simulink model "DogGait_Sine"  (R2022b)
settings: Solver=FixedStepAuto  StartTime=0.0  StopTime=inf  RelTol=1e-3
undefined symbols (not defined in the file): C, D, f
libraries: vexv5lib x24, vexcommonlib x16, Vex_V5_Simulink_Expansion x8
settings Model: Creator=Serious Chimp  LastModifiedBy=Serious Chimp
settings DataIOCC: SaveFormat=StructureWithTime  InspectSignalLogs=on
settings OptimizationCC: EnhancedBackFolding=on  PassReuseOutputArgsAs=Individual arguments  ZeroExternalMemoryAtStartup=off  ZeroInternalMemoryAtStartup=off  MaxStackSize=64  OptimizeBlockOrder=speed  DifferentSizesBufferReuse=on  OptimizationCustomize=off  EfficientTunableParamExpr=on
settings DebuggingCC: ParameterTunabilityLossMsg=error
settings HardwareCC: ProdBitPerPointer=32  ProdBitPerSizeT=32  ProdBitPerPtrDiffT=32  ProdLargestAtomicInteger=Long  ProdLargestAtomicFloat=Double  ProdWordSize=32  ProdHWDeviceType=ARM Compatible->ARM Cortex  UseEmbeddedCoderFeatures=off
settings SFSimCC: MATLABDynamicMemAlloc=off
settings RTWCC: Description=Embedded Coder  SystemTargetFile=ert.tlc  HardwareBoard=VEX V5 Robot Brain  TLCOptions="-aInlineSetEventsForThisBaseRateFcn=TLC_FALSE -aSuppressMultiTaskScheduler=TLC_FALSE  -aRateBasedStepFcn=0"  TemplateMakefile=ert_default_tmf  Toolchain=GNU Tools for ARM Embedded Processors
settings CodeAppCC: ForceParamTrailComments=on  IgnoreCustomStorageClasses=off  OperatorAnnotations=on  SimulinkDataObjDesc=on  SFDataObjDesc=on  InsertBlockDesc=on
settings ERTTargetCC: SupportNonInlinedSFcns=on  ExtModeTransport=3  ExtModeStaticAlloc=on  ExtModeStaticAllocSize=2048  ExtModeMexFile=ext_xcp  ExtModeIntrfLevel=Level2 - Open

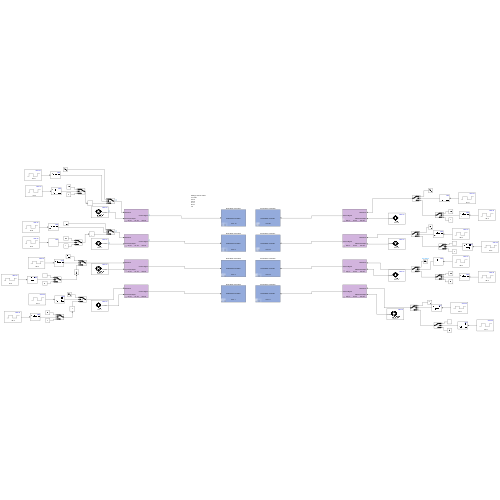
[thumbnail: Simulink's stored preview of the top-level diagram]
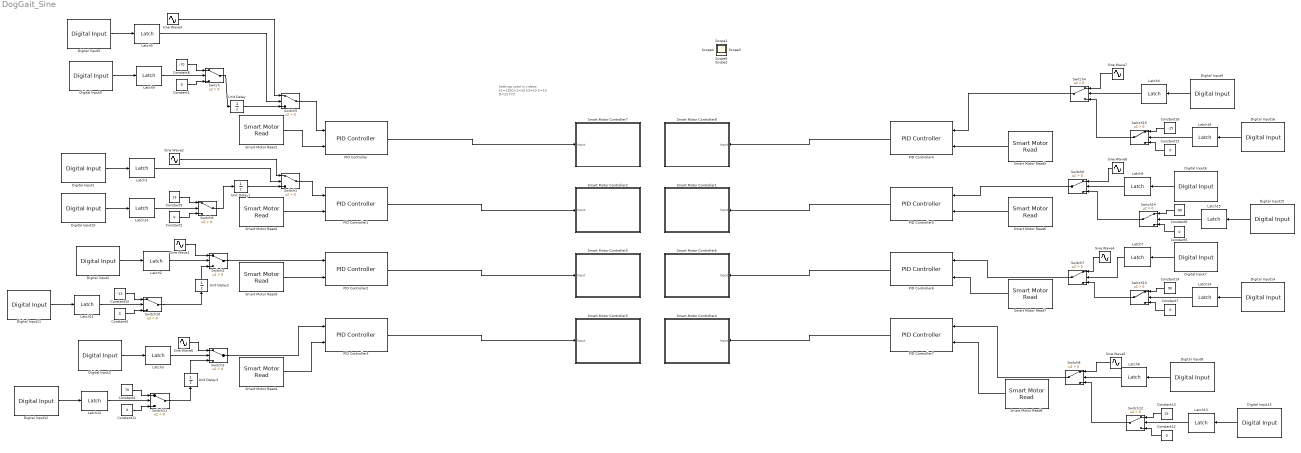
== system DogGait_Sine ==
  note: Settings used in videos:
      | k1=1200
      | k2=10
      | k3=10
      | C=15
      | D=23
      | f=5
  Constant{1..3,5,7,11..12,15} (8 alike) : Constant  Value=0
  Constant10 : Constant  Value=-13
  Constant13 : Constant  Value=15
  Constant14 : Constant  Value=90
  Constant16 : Constant  Value=-15
  Constant4 : Constant  Value=70
  Constant6 : Constant  Value=-90
  Constant8 : Constant  Value=-70
  Constant9 : Constant  Value=13
  Digital Input{1..8} (8 alike) : vexv5lib/Sensors/Digital Input  smartPort3wire=None  port=H  SampleTime=0.2
  Digital Input{9..16} (8 alike) : vexv5lib/Sensors/Digital Input  smartPort3wire=None  port=A  SampleTime=0.2
  Latch{1..16} (16 alike) : vexcommonlib/Latch  output0=off  BlockPlatform=vexv5
      settings: LibrarySourceBlock=vexv5lib/Utilities/Latch
  PID Controller : Vex_V5_Simulink_Expansion/Core Blocks/PID Controller  KP=k1  KI=k3  KD=k2  LimitOutput=off  limitHigh=10  limitLow=10  AntiWindupMode=none  kb=0
      settings: SourceProductName=Vex V5 Simulink Expansion
  PID Controller{1..7} (7 alike) : Vex_V5_Simulink_Expansion/Core Blocks/PID Controller  KP=k1  KI=k3  KD=k2  LimitOutput=off  limitHigh=0  limitLow=0  AntiWindupMode=none  kb=0
      settings: SourceProductName=Vex V5 Simulink Expansion
  Sine Wave1 : Sin  Amplitude=-C  Bias=-13  Frequency=f  SampleTime=1e-3
  Sine Wave2 : Sin  Amplitude=-C  Bias=13  Frequency=f  SampleTime=1e-3
  Sine Wave3 : Sin  Amplitude=D  Bias=-70  Frequency=f  Phase=-f/2  SampleTime=1e-3
  Sine Wave4 : Sin  Amplitude=D  Bias=90  Frequency=f  SampleTime=1e-3
  Sine Wave5 : Sin  Amplitude=-C  Bias=15  Frequency=f  Phase=f/2  SampleTime=1e-3
  Sine Wave6 : Sin  Amplitude=D  Bias=70  Frequency=f  Phase=-f/2  SampleTime=1e-3
  Sine Wave7 : Sin  Amplitude=-C  Bias=-15  Frequency=f  Phase=f/2  SampleTime=1e-3
  Sine Wave8 : Sin  Amplitude=D  Bias=-90  Frequency=f  SampleTime=1e-3
  Smart Motor Controller1 : Subsystem  AncestorBlock=Vex_V5_Simulink_Expansion/Core Blocks/Smart Motor Controller  mask(Smart Motor Controller){motorPort=19, OperationMode=Advanced Control, MotorBrakeMode=Coast}
      mask prompts: motorPort "Smart Port:"; OperationMode "Control Mode:"; MotorBrakeMode "Braking Mode:"
      mask help: Controls the Vex Smart Motor via the chosen method.
      mask TypeOptions motorPort: Advanced_SmartMotorWrite/motorPort
      mask TypeOptions OperationMode: Advanced_SmartMotorWrite/OperationMode
      mask TypeOptions MotorBrakeMode: Advanced_SmartMotorWrite/MotorBrakeMode
      mask DialogControl Container3 Prompt: Smart Motor Configuration
      mask Display:
      | %mode = get_param(gcb, 'control');
      | port = get_param(gcb, 'motorPort');
      | %text(0.3,0.45,[mode]);
      | 
      | text(0.5,0.5, 'Smart Motor Controller','HorizontalAlignment','center');
      | text(0.42,0.15, ['Port: ',port]);
  Smart Motor Controller2 : Subsystem  AncestorBlock=Vex_V5_Simulink_Expansion/Core Blocks/Smart Motor Controller  mask(Smart Motor Controller){motorPort=9, OperationMode=Advanced Control, MotorBrakeMode=Coast}
      mask prompts: motorPort "Smart Port:"; OperationMode "Control Mode:"; MotorBrakeMode "Braking Mode:"
      mask help: Controls the Vex Smart Motor via the chosen method.
      mask TypeOptions motorPort: Advanced_SmartMotorWrite/motorPort
      mask TypeOptions OperationMode: Advanced_SmartMotorWrite/OperationMode
      mask TypeOptions MotorBrakeMode: Advanced_SmartMotorWrite/MotorBrakeMode
      mask DialogControl Container3 Prompt: Smart Motor Configuration
      mask Display:
      | %mode = get_param(gcb, 'control');
      | port = get_param(gcb, 'motorPort');
      | %text(0.3,0.45,[mode]);
      | 
      | text(0.5,0.5, 'Smart Motor Controller','HorizontalAlignment','center');
      | text(0.42,0.15, ['Port: ',port]);
  Smart Motor Controller3 : Subsystem  AncestorBlock=Vex_V5_Simulink_Expansion/Core Blocks/Smart Motor Controller  mask(Smart Motor Controller){motorPort=1, OperationMode=Advanced Control, MotorBrakeMode=Coast}
      mask prompts: motorPort "Smart Port:"; OperationMode "Control Mode:"; MotorBrakeMode "Braking Mode:"
      mask help: Controls the Vex Smart Motor via the chosen method.
      mask TypeOptions motorPort: Advanced_SmartMotorWrite/motorPort
      mask TypeOptions OperationMode: Advanced_SmartMotorWrite/OperationMode
      mask TypeOptions MotorBrakeMode: Advanced_SmartMotorWrite/MotorBrakeMode
      mask DialogControl Container3 Prompt: Smart Motor Configuration
      mask Display:
      | %mode = get_param(gcb, 'control');
      | port = get_param(gcb, 'motorPort');
      | %text(0.3,0.45,[mode]);
      | 
      | text(0.5,0.5, 'Smart Motor Controller','HorizontalAlignment','center');
      | text(0.42,0.15, ['Port: ',port]);
  Smart Motor Controller4 : Subsystem  AncestorBlock=Vex_V5_Simulink_Expansion/Core Blocks/Smart Motor Controller  mask(Smart Motor Controller){motorPort=11, OperationMode=Advanced Control, MotorBrakeMode=Coast}
      mask prompts: motorPort "Smart Port:"; OperationMode "Control Mode:"; MotorBrakeMode "Braking Mode:"
      mask help: Controls the Vex Smart Motor via the chosen method.
      mask TypeOptions motorPort: Advanced_SmartMotorWrite/motorPort
      mask TypeOptions OperationMode: Advanced_SmartMotorWrite/OperationMode
      mask TypeOptions MotorBrakeMode: Advanced_SmartMotorWrite/MotorBrakeMode
      mask DialogControl Container3 Prompt: Smart Motor Configuration
      mask Display:
      | %mode = get_param(gcb, 'control');
      | port = get_param(gcb, 'motorPort');
      | %text(0.3,0.45,[mode]);
      | 
      | text(0.5,0.5, 'Smart Motor Controller','HorizontalAlignment','center');
      | text(0.42,0.15, ['Port: ',port]);
  Smart Motor Controller5 : Subsystem  AncestorBlock=Vex_V5_Simulink_Expansion/Core Blocks/Smart Motor Controller  mask(Smart Motor Controller){motorPort=2, OperationMode=Advanced Control, MotorBrakeMode=Coast}
      mask prompts: motorPort "Smart Port:"; OperationMode "Control Mode:"; MotorBrakeMode "Braking Mode:"
      mask help: Controls the Vex Smart Motor via the chosen method.
      mask TypeOptions motorPort: Advanced_SmartMotorWrite/motorPort
      mask TypeOptions OperationMode: Advanced_SmartMotorWrite/OperationMode
      mask TypeOptions MotorBrakeMode: Advanced_SmartMotorWrite/MotorBrakeMode
      mask DialogControl Container3 Prompt: Smart Motor Configuration
      mask Display:
      | %mode = get_param(gcb, 'control');
      | port = get_param(gcb, 'motorPort');
      | %text(0.3,0.45,[mode]);
      | 
      | text(0.5,0.5, 'Smart Motor Controller','HorizontalAlignment','center');
      | text(0.42,0.15, ['Port: ',port]);
  Smart Motor Controller6 : Subsystem  AncestorBlock=Vex_V5_Simulink_Expansion/Core Blocks/Smart Motor Controller  mask(Smart Motor Controller){motorPort=12, OperationMode=Advanced Control, MotorBrakeMode=Coast}
      mask prompts: motorPort "Smart Port:"; OperationMode "Control Mode:"; MotorBrakeMode "Braking Mode:"
      mask help: Controls the Vex Smart Motor via the chosen method.
      mask TypeOptions motorPort: Advanced_SmartMotorWrite/motorPort
      mask TypeOptions OperationMode: Advanced_SmartMotorWrite/OperationMode
      mask TypeOptions MotorBrakeMode: Advanced_SmartMotorWrite/MotorBrakeMode
      mask DialogControl Container3 Prompt: Smart Motor Configuration
      mask Display:
      | %mode = get_param(gcb, 'control');
      | port = get_param(gcb, 'motorPort');
      | %text(0.3,0.45,[mode]);
      | 
      | text(0.5,0.5, 'Smart Motor Controller','HorizontalAlignment','center');
      | text(0.42,0.15, ['Port: ',port]);
  Smart Motor Controller7 : Subsystem  AncestorBlock=Vex_V5_Simulink_Expansion/Core Blocks/Smart Motor Controller  mask(Smart Motor Controller){motorPort=10, OperationMode=Advanced Control, MotorBrakeMode=Coast}
      mask prompts: motorPort "Smart Port:"; OperationMode "Control Mode:"; MotorBrakeMode "Braking Mode:"
      mask help: Controls the Vex Smart Motor via the chosen method.
      mask TypeOptions motorPort: Advanced_SmartMotorWrite/motorPort
      mask TypeOptions OperationMode: Advanced_SmartMotorWrite/OperationMode
      mask TypeOptions MotorBrakeMode: Advanced_SmartMotorWrite/MotorBrakeMode
      mask DialogControl Container3 Prompt: Smart Motor Configuration
      mask Display:
      | %mode = get_param(gcb, 'control');
      | port = get_param(gcb, 'motorPort');
      | %text(0.3,0.45,[mode]);
      | 
      | text(0.5,0.5, 'Smart Motor Controller','HorizontalAlignment','center');
      | text(0.42,0.15, ['Port: ',port]);
  Smart Motor Controller8 : Subsystem  AncestorBlock=Vex_V5_Simulink_Expansion/Core Blocks/Smart Motor Controller  mask(Smart Motor Controller){motorPort=20, OperationMode=Advanced Control, MotorBrakeMode=Coast}
      mask prompts: motorPort "Smart Port:"; OperationMode "Control Mode:"; MotorBrakeMode "Braking Mode:"
      mask help: Controls the Vex Smart Motor via the chosen method.
      mask TypeOptions motorPort: Advanced_SmartMotorWrite/motorPort
      mask TypeOptions OperationMode: Advanced_SmartMotorWrite/OperationMode
      mask TypeOptions MotorBrakeMode: Advanced_SmartMotorWrite/MotorBrakeMode
      mask DialogControl Container3 Prompt: Smart Motor Configuration
      mask Display:
      | %mode = get_param(gcb, 'control');
      | port = get_param(gcb, 'motorPort');
      | %text(0.3,0.45,[mode]);
      | 
      | text(0.5,0.5, 'Smart Motor Controller','HorizontalAlignment','center');
      | text(0.42,0.15, ['Port: ',port]);
  Smart Motor Read1 : vexv5lib/Sensors/Smart Motor Read  motorPort=10  EncoderUnit=Degrees  resetOption=No reset  additionalOutput=off  SampleTime=0.01
  Smart Motor Read2 : vexv5lib/Sensors/Smart Motor Read  motorPort=9  EncoderUnit=Degrees  resetOption=No reset  additionalOutput=off  SampleTime=0.01
  Smart Motor Read3 : vexv5lib/Sensors/Smart Motor Read  motorPort=2  EncoderUnit=Degrees  resetOption=No reset  additionalOutput=off  SampleTime=0.01
  Smart Motor Read4 : vexv5lib/Sensors/Smart Motor Read  motorPort=1  EncoderUnit=Degrees  resetOption=No reset  additionalOutput=off  SampleTime=0.01
  Smart Motor Read5 : vexv5lib/Sensors/Smart Motor Read  motorPort=20  EncoderUnit=Degrees  resetOption=No reset  additionalOutput=off  SampleTime=0.01
  Smart Motor Read6 : vexv5lib/Sensors/Smart Motor Read  motorPort=19  EncoderUnit=Degrees  resetOption=No reset  additionalOutput=off  SampleTime=0.01
  Smart Motor Read7 : vexv5lib/Sensors/Smart Motor Read  motorPort=12  EncoderUnit=Degrees  resetOption=No reset  additionalOutput=off  SampleTime=0.01
  Smart Motor Read8 : vexv5lib/Sensors/Smart Motor Read  motorPort=11  EncoderUnit=Degrees  resetOption=No reset  additionalOutput=off  SampleTime=0.01
  Switch{,1..15} (16 alike) : Switch  Criteria=u2 > Threshold  SaturateOnIntegerOverflow=off  InputSameDT=off
  Unit Delay{,1..3} (4 alike) : UnitDelay  SampleTime=-1  HasFrameUpgradeWarning=on
  Scope{,1..5} (6 alike) : Scope
  wires:
  Smart Motor Read1/1 -> PID Controller/2
  Smart Motor Read2/1 -> PID Controller1/2
  Smart Motor Read4/1 -> PID Controller3/2
  Smart Motor Read3/1 -> PID Controller2/2
  Smart Motor Read5/1 -> PID Controller4/2
  Smart Motor Read6/1 -> PID Controller5/2
  Smart Motor Read7/1 -> PID Controller6/2
  Smart Motor Read8/1 -> PID Controller7/2
  Sine Wave3/1 -> Switch5/1
  Sine Wave5/1 -> Switch8/1
  Sine Wave7/1 -> Switch4/1
  Sine Wave2/1 -> Switch1/1
  Sine Wave1/1 -> Switch2/1
  Sine Wave4/1 -> Switch7/1
  Sine Wave6/1 -> Switch3/1
  Sine Wave8/1 -> Switch6/1
  Digital Input5/1 -> Latch5/1
  Latch5/1 -> Switch5/2
  Switch5/1 -> PID Controller/1
  Switch9/1 -> Unit Delay1/1
  Digital Input1/1 -> Latch1/1
  Latch1/1 -> Switch1/2
  Switch1/1 -> PID Controller1/1
  Digital Input2/1 -> Latch2/1
  Latch2/1 -> Switch2/2
  Switch2/1 -> PID Controller2/1
  Digital Input3/1 -> Latch3/1
  Latch3/1 -> Switch3/2
  Switch3/1 -> PID Controller3/1
  Digital Input4/1 -> Latch4/1
  Latch4/1 -> Switch4/2
  Switch4/1 -> PID Controller4/1
  Digital Input6/1 -> Latch6/1
  Latch6/1 -> Switch6/2
  Switch6/1 -> PID Controller5/1
  Digital Input7/1 -> Latch7/1
  Latch7/1 -> Switch7/2
  Switch7/1 -> PID Controller6/1
  Digital Input8/1 -> Latch8/1
  Latch8/1 -> Switch8/2
  Switch8/1 -> PID Controller7/1
  Constant1/1 -> Switch/3
  Constant8/1 -> Switch/1
  Digital Input9/1 -> Latch9/1
  Latch9/1 -> Switch/2
  Constant9/1 -> Switch9/1
  Latch10/1 -> Switch9/2
  Constant2/1 -> Switch9/3
  Digital Input10/1 -> Latch10/1
  Constant10/1 -> Switch10/1
  Latch11/1 -> Switch10/2
  Constant3/1 -> Switch10/3
  Digital Input11/1 -> Latch11/1
  Constant11/1 -> Switch11/3
  Constant4/1 -> Switch11/1
  Digital Input12/1 -> Latch12/1
  Latch12/1 -> Switch11/2
  Digital Input13/1 -> Latch13/1
  Constant13/1 -> Switch12/1
  Constant12/1 -> Switch12/3
  Latch13/1 -> Switch12/2
  Digital Input14/1 -> Latch14/1
  Constant14/1 -> Switch13/1
  Constant7/1 -> Switch13/3
  Latch14/1 -> Switch13/2
  Digital Input15/1 -> Latch15/1
  Constant6/1 -> Switch14/1
  Constant5/1 -> Switch14/3
  Latch15/1 -> Switch14/2
  Digital Input16/1 -> Latch16/1
  Constant16/1 -> Switch15/1
  Constant15/1 -> Switch15/3
  Latch16/1 -> Switch15/2
  Switch/1 -> Unit Delay/1
  Switch10/1 -> Unit Delay2/1
  Unit Delay2/1 -> Switch2/3
  Unit Delay1/1 -> Switch1/3
  Unit Delay/1 -> Switch5/3
  Switch13/1 -> Switch7/3
  Switch14/1 -> Switch6/3
  Unit Delay3/1 -> Switch3/3
  Switch11/1 -> Unit Delay3/1
  Switch15/1 -> Switch4/3
  Switch12/1 -> Switch8/3
  PID Controller/1 -> Smart Motor Controller7/1(" Input")
  PID Controller1/1 -> Smart Motor Controller2/1(" Input")
  PID Controller2/1 -> Smart Motor Controller5/1(" Input")
  PID Controller3/1 -> Smart Motor Controller3/1(" Input")
  PID Controller4/1 -> Smart Motor Controller8/1(" Input")
  PID Controller5/1 -> Smart Motor Controller1/1(" Input")
  PID Controller6/1 -> Smart Motor Controller6/1(" Input")
  PID Controller7/1 -> Smart Motor Controller4/1(" Input")

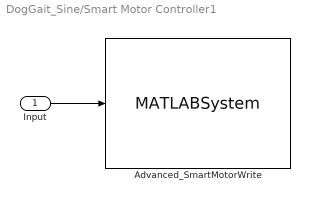
== system DogGait_Sine/Smart Motor Controller1 ==
  " Input" : Inport
  Advanced_SmartMotorWrite : MATLABSystem  System=Advanced_SmartMotorWrite  motorPort=19  scaleFactor=36:1  MotorBrakeMode=Coast  OperationMode=Advanced Control
      mask Type: Advanced_SmartMotorWrite
      mask Display:
      | color('white');
      | plot([100,100,100,100]*1,[100,100,100,100]*1);
      | plot([100,100,100,100]*0,[100,100,100,100]*0);
      | color('black');
      | image(fullfile(codertarget.vexv5.internal.getSpPkgRootDir, 'resources', 'vex-v5-motor2.png'),'center');
      | patch([0.8, 0.8, 1, 1], [0.82857, 1, 1, 0.82857], [1, 1, 1]);
      | color('blue');
      | text(99, 92, 'VEX V5 ', 'horizontalAlignment', 'right');
      | color('black');
      | text(62,12,'Port: 19','horizontalAlignment','center');
      | 
      | port_label('Input',1,'Voltage(mV)');
  wires:
  " Input"/1 -> Advanced_SmartMotorWrite/1

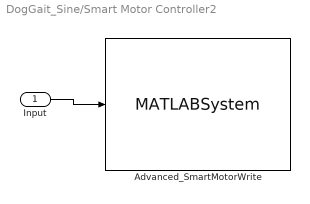
== system DogGait_Sine/Smart Motor Controller2 ==
  " Input" : Inport
  Advanced_SmartMotorWrite : MATLABSystem  System=Advanced_SmartMotorWrite  motorPort=9  scaleFactor=36:1  MotorBrakeMode=Coast  OperationMode=Advanced Control
      mask Type: Advanced_SmartMotorWrite
      mask Display:
      | color('white');
      | plot([100,100,100,100]*1,[100,100,100,100]*1);
      | plot([100,100,100,100]*0,[100,100,100,100]*0);
      | color('black');
      | image(fullfile(codertarget.vexv5.internal.getSpPkgRootDir, 'resources', 'vex-v5-motor2.png'),'center');
      | patch([0.8, 0.8, 1, 1], [0.82857, 1, 1, 0.82857], [1, 1, 1]);
      | color('blue');
      | text(99, 92, 'VEX V5 ', 'horizontalAlignment', 'right');
      | color('black');
      | text(62,12,'Port: 9','horizontalAlignment','center');
      | 
      | port_label('Input',1,'Voltage(mV)');
  wires:
  " Input"/1 -> Advanced_SmartMotorWrite/1

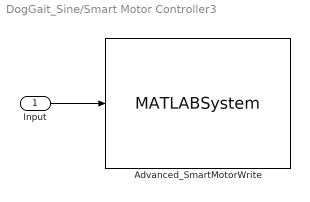
== system DogGait_Sine/Smart Motor Controller3 ==
  " Input" : Inport
  Advanced_SmartMotorWrite : MATLABSystem  System=Advanced_SmartMotorWrite  motorPort=1  scaleFactor=36:1  MotorBrakeMode=Coast  OperationMode=Advanced Control
      mask Type: Advanced_SmartMotorWrite
      mask Display:
      | color('white');
      | plot([100,100,100,100]*1,[100,100,100,100]*1);
      | plot([100,100,100,100]*0,[100,100,100,100]*0);
      | color('black');
      | image(fullfile(codertarget.vexv5.internal.getSpPkgRootDir, 'resources', 'vex-v5-motor2.png'),'center');
      | patch([0.8, 0.8, 1, 1], [0.82857, 1, 1, 0.82857], [1, 1, 1]);
      | color('blue');
      | text(99, 92, 'VEX V5 ', 'horizontalAlignment', 'right');
      | color('black');
      | text(62,12,'Port: 1','horizontalAlignment','center');
      | 
      | port_label('Input',1,'Voltage(mV)');
  wires:
  " Input"/1 -> Advanced_SmartMotorWrite/1

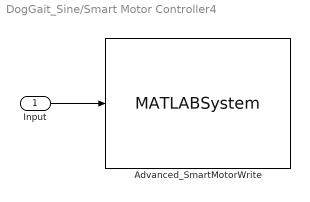
== system DogGait_Sine/Smart Motor Controller4 ==
  " Input" : Inport
  Advanced_SmartMotorWrite : MATLABSystem  System=Advanced_SmartMotorWrite  motorPort=11  scaleFactor=36:1  MotorBrakeMode=Coast  OperationMode=Advanced Control
      mask Type: Advanced_SmartMotorWrite
      mask Display:
      | color('white');
      | plot([100,100,100,100]*1,[100,100,100,100]*1);
      | plot([100,100,100,100]*0,[100,100,100,100]*0);
      | color('black');
      | image(fullfile(codertarget.vexv5.internal.getSpPkgRootDir, 'resources', 'vex-v5-motor2.png'),'center');
      | patch([0.8, 0.8, 1, 1], [0.82857, 1, 1, 0.82857], [1, 1, 1]);
      | color('blue');
      | text(99, 92, 'VEX V5 ', 'horizontalAlignment', 'right');
      | color('black');
      | text(62,12,'Port: 11','horizontalAlignment','center');
      | 
      | port_label('Input',1,'Voltage(mV)');
  wires:
  " Input"/1 -> Advanced_SmartMotorWrite/1

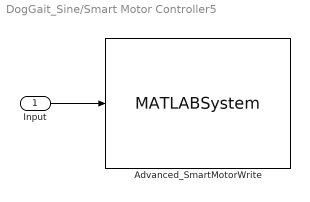
== system DogGait_Sine/Smart Motor Controller5 ==
  " Input" : Inport
  Advanced_SmartMotorWrite : MATLABSystem  System=Advanced_SmartMotorWrite  motorPort=2  scaleFactor=36:1  MotorBrakeMode=Coast  OperationMode=Advanced Control
      mask Type: Advanced_SmartMotorWrite
      mask Display:
      | color('white');
      | plot([100,100,100,100]*1,[100,100,100,100]*1);
      | plot([100,100,100,100]*0,[100,100,100,100]*0);
      | color('black');
      | image(fullfile(codertarget.vexv5.internal.getSpPkgRootDir, 'resources', 'vex-v5-motor2.png'),'center');
      | patch([0.8, 0.8, 1, 1], [0.82857, 1, 1, 0.82857], [1, 1, 1]);
      | color('blue');
      | text(99, 92, 'VEX V5 ', 'horizontalAlignment', 'right');
      | color('black');
      | text(62,12,'Port: 2','horizontalAlignment','center');
      | 
      | port_label('Input',1,'Voltage(mV)');
  wires:
  " Input"/1 -> Advanced_SmartMotorWrite/1

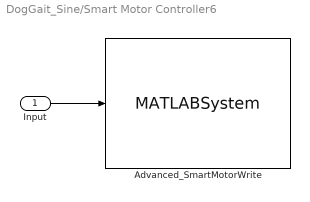
== system DogGait_Sine/Smart Motor Controller6 ==
  " Input" : Inport
  Advanced_SmartMotorWrite : MATLABSystem  System=Advanced_SmartMotorWrite  motorPort=12  scaleFactor=36:1  MotorBrakeMode=Coast  OperationMode=Advanced Control
      mask Type: Advanced_SmartMotorWrite
      mask Display:
      | color('white');
      | plot([100,100,100,100]*1,[100,100,100,100]*1);
      | plot([100,100,100,100]*0,[100,100,100,100]*0);
      | color('black');
      | image(fullfile(codertarget.vexv5.internal.getSpPkgRootDir, 'resources', 'vex-v5-motor2.png'),'center');
      | patch([0.8, 0.8, 1, 1], [0.82857, 1, 1, 0.82857], [1, 1, 1]);
      | color('blue');
      | text(99, 92, 'VEX V5 ', 'horizontalAlignment', 'right');
      | color('black');
      | text(62,12,'Port: 12','horizontalAlignment','center');
      | 
      | port_label('Input',1,'Voltage(mV)');
  wires:
  " Input"/1 -> Advanced_SmartMotorWrite/1

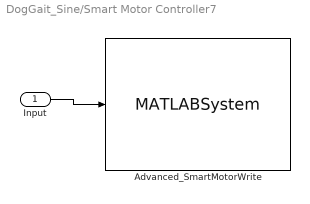
== system DogGait_Sine/Smart Motor Controller7 ==
  " Input" : Inport
  Advanced_SmartMotorWrite : MATLABSystem  System=Advanced_SmartMotorWrite  motorPort=10  scaleFactor=36:1  MotorBrakeMode=Coast  OperationMode=Advanced Control
      mask Type: Advanced_SmartMotorWrite
      mask Display:
      | color('white');
      | plot([100,100,100,100]*1,[100,100,100,100]*1);
      | plot([100,100,100,100]*0,[100,100,100,100]*0);
      | color('black');
      | image(fullfile(codertarget.vexv5.internal.getSpPkgRootDir, 'resources', 'vex-v5-motor2.png'),'center');
      | patch([0.8, 0.8, 1, 1], [0.82857, 1, 1, 0.82857], [1, 1, 1]);
      | color('blue');
      | text(99, 92, 'VEX V5 ', 'horizontalAlignment', 'right');
      | color('black');
      | text(62,12,'Port: 10','horizontalAlignment','center');
      | 
      | port_label('Input',1,'Voltage(mV)');
  wires:
  " Input"/1 -> Advanced_SmartMotorWrite/1

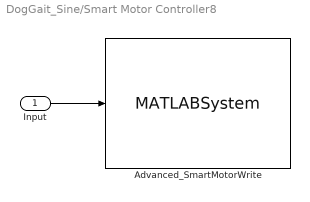
== system DogGait_Sine/Smart Motor Controller8 ==
  " Input" : Inport
  Advanced_SmartMotorWrite : MATLABSystem  System=Advanced_SmartMotorWrite  motorPort=20  scaleFactor=36:1  MotorBrakeMode=Coast  OperationMode=Advanced Control
      mask Type: Advanced_SmartMotorWrite
      mask Display:
      | color('white');
      | plot([100,100,100,100]*1,[100,100,100,100]*1);
      | plot([100,100,100,100]*0,[100,100,100,100]*0);
      | color('black');
      | image(fullfile(codertarget.vexv5.internal.getSpPkgRootDir, 'resources', 'vex-v5-motor2.png'),'center');
      | patch([0.8, 0.8, 1, 1], [0.82857, 1, 1, 0.82857], [1, 1, 1]);
      | color('blue');
      | text(99, 92, 'VEX V5 ', 'horizontalAlignment', 'right');
      | color('black');
      | text(62,12,'Port: 20','horizontalAlignment','center');
      | 
      | port_label('Input',1,'Voltage(mV)');
  wires:
  " Input"/1 -> Advanced_SmartMotorWrite/1
